simulink model "empirical_cell_twaice_balancing"  (R2024b)
settings: Solver=FixedStepAuto  StartTime=0.0  StopTime=inf  FixedStep=1  RelTol=1e-3
values from neighbouring files (symbols this model uses):
  act = 1    [RunMe_TWAICE_Cell_Model_Farasis_P75_75Ah_v8_1_3.m]
  lic_no = fin_convert(Prod_lic)    [RunMe_TWAICE_Cell_Model_Farasis_P75_75Ah_v8_1_3.m]
  Ts = 1    [RunMe_TWAICE_Cell_Model_Farasis_P75_75Ah_v8_1_3.m]
undefined symbols (not defined in the file or in its folder): DWORK0, DWORK1, DWORK10, DWORK11, DWORK12, DWORK13, DWORK14, DWORK15, DWORK16, DWORK17, DWORK18, DWORK19, DWORK2, DWORK20, DWORK22, DWORK23, DWORK24, DWORK25, DWORK26, DWORK27, DWORK28, DWORK29, DWORK3, DWORK30, DWORK31, DWORK32, DWORK33, DWORK34, DWORK35, DWORK36, DWORK4, DWORK5, DWORK6, DWORK7, DWORK8, DWORK9, SOHc_init, SOHr_init
libraries: fl_lib x73, nesl_utility x32, ee_lib x8
(part 3 of 4)

== system empirical_cell_twaice_balancing/Cell 5/ETA Model 1 ==
  "Current " : Inport  OutDataTypeStr=double  PortDimensions=1
  T_ambient / °C : Inport  Port=2  OutDataTypeStr=double  PortDimensions=1
  SOHc_init : Inport  Port=3
  SOHr_init : Inport  Port=4
  SOC_init : Inport  Port=5
  T_init : Inport  Port=6
  SOC_in : Inport  Port=7
  SOH : Inport  Port=8
  ETA Model _sfcn : S-Function  FunctionName=ETA_sf  Parameters=sfcnParam1, sfcnParam2, sfcnParam3  SFunctionModules=""  SFunctionDeploymentMode=off  EnableBusSupport=off  SFcnStateName=DWORK0,DWORK1,DWORK2,DWORK3,DWORK4,DWORK5,DWORK6,DWORK7,DWORK8,DWORK9,DWORK10,DWORK11,DWORK12,DWORK13,DWORK14,DWORK15,DWORK16,DWORK17,DWORK18,DWORK19,DWORK20,DWORK22,DWORK23,DWORK24,DWORK25,DWORK26,DWORK27,DWORK28,DWORK29,DWORK30,DWORK31,DWORK32,DWORK33,DWORK34,DWORK35,DWORK36  mask{rtw_sf_name=ETA_sf, showVar=off, sfcnParam1=sfcnParam1, sfcnParam2=sfcnParam2, sfcnParam3=sfcnParam3}
      mask prompts: rtw_sf_name "Simulink:masks:GenSFuncName_MP"; showVar "Simulink:masks:GenSFuncShowModuleList_MP"; sfcnParam1 "Ts:"; sfcnParam2 "act:"; sfcnParam3 "lic_no:"
      mask help: Simulink:masks:GenSFuncDesc_MD
      mask init: same as empirical_cell_twaice_balancing/Cell 1/ETA Model 1/ETA Model _sfcn
      settings: SFcnIsStateOwnerBlock=on
      settings: CopyFcn=|
      | if ~strcmp(get_param(gcb,'Linkstatus'),'none') && ...
      | ~strcmp(get_param(gcb,'Linkstatus'),'implicit')
      |   set_param(gcb,'LinkStatus','none');
      | end
      mask Help: eval('feval(''rtwprivate'',''rtwhelpview'',''rtw_sfcn_block'')');
      mask Display:
      | port_label('input',1,'Current ');
      | port_label('input',2,'T_ambient / °C');
      | port_label('input',3,'htc_in');
      | port_label('input',4,'Pcool_in');
      | port_label('input',5,'SOHc_init');
      | port_label('input',6,'SOHr_init');
      | port_label('input',7,'SOC_init');
      | port_label('input',8,'T_init');
      | port_label('input',9,'SOC_in');
      | port_label('input',10,'SOHc');
      | port_label('input',11,'SOHr');
      | port_label('output',1,'Current / A');
      | port_label('output',2,'Voltage / V');
      | port_label('output',3,'SOC / 0..1');
      | port_label('output',4,'SOHc / 0..1');
      | port_label('output',5,'T_sim / °C');
      | port_label('output',6,'Generated Heat / W');
      | port_label('output',7,'SOHr / 1');
      | port_label('output',8,'Power_sim / W');
      | port_label('output',9,'total_Ah');
  __InputSSForSFun__ : Subsystem
  __OutputSSForSFun__ : Subsystem
  Current / A : Outport  OutDataTypeStr=double  PortDimensions=1
  Voltage / V : Outport  Port=2  OutDataTypeStr=double  PortDimensions=1
  SOC / 0..1 : Outport  Port=3  OutDataTypeStr=double  PortDimensions=1
  SOHc / 0..1 : Outport  Port=4  OutDataTypeStr=double  PortDimensions=1
  T_sim / °C : Outport  Port=5  OutDataTypeStr=double  PortDimensions=1
  Generated Heat / W : Outport  Port=6  OutDataTypeStr=double  PortDimensions=1
  SOHr / 1 : Outport  Port=7  OutDataTypeStr=double  PortDimensions=1
  Power_sim / W : Outport  Port=8  OutDataTypeStr=double  PortDimensions=1
  total_Ah : Outport  Port=9
  wires:
  "Current "/1 -> __InputSSForSFun__/1("Current ")
  T_ambient / °C/1 -> __InputSSForSFun__/2(T_ambient / °C)
  SOHc_init/1 -> __InputSSForSFun__/3(SOHc_init)
  SOHr_init/1 -> __InputSSForSFun__/4(SOHr_init)
  SOC_init/1 -> __InputSSForSFun__/5(SOC_init)
  T_init/1 -> __InputSSForSFun__/6(T_init)
  SOC_in/1 -> __InputSSForSFun__/7(SOC_in)
  SOH/1 -> __InputSSForSFun__/8(SOH)
  __InputSSForSFun__/1(__UniqueOutportName__1__) -> ETA Model _sfcn/1
  __InputSSForSFun__/2(__UniqueOutportName__2__) -> ETA Model _sfcn/2
  __InputSSForSFun__/3(__UniqueOutportName__3__) -> ETA Model _sfcn/3
  __InputSSForSFun__/4(__UniqueOutportName__4__) -> ETA Model _sfcn/4
  __InputSSForSFun__/5(__UniqueOutportName__5__) -> ETA Model _sfcn/5
  __InputSSForSFun__/6(__UniqueOutportName__6__) -> ETA Model _sfcn/6
  __InputSSForSFun__/7(__UniqueOutportName__7__) -> ETA Model _sfcn/7
  __InputSSForSFun__/8(__UniqueOutportName__8__) -> ETA Model _sfcn/8
  __InputSSForSFun__/9(__UniqueOutportName__9__) -> ETA Model _sfcn/9
  __InputSSForSFun__/10(__UniqueOutportName__10__) -> ETA Model _sfcn/10
  __InputSSForSFun__/11(__UniqueOutportName__11__) -> ETA Model _sfcn/11
  ETA Model _sfcn/1 -> __OutputSSForSFun__/1(__UniqueInportName__1__)
  ETA Model _sfcn/2 -> __OutputSSForSFun__/2(__UniqueInportName__2__)
  ETA Model _sfcn/3 -> __OutputSSForSFun__/3(__UniqueInportName__3__)
  ETA Model _sfcn/4 -> __OutputSSForSFun__/4(__UniqueInportName__4__)
  ETA Model _sfcn/5 -> __OutputSSForSFun__/5(__UniqueInportName__5__)
  ETA Model _sfcn/6 -> __OutputSSForSFun__/6(__UniqueInportName__6__)
  ETA Model _sfcn/7 -> __OutputSSForSFun__/7(__UniqueInportName__7__)
  ETA Model _sfcn/8 -> __OutputSSForSFun__/8(__UniqueInportName__8__)
  ETA Model _sfcn/9 -> __OutputSSForSFun__/9(__UniqueInportName__9__)
  __OutputSSForSFun__/1(Current / A) -> Current / A/1
  __OutputSSForSFun__/2(Voltage / V) -> Voltage / V/1
  __OutputSSForSFun__/3(SOC / 0..1) -> SOC / 0..1/1
  __OutputSSForSFun__/4(SOHc / 0..1) -> SOHc / 0..1/1
  __OutputSSForSFun__/5(T_sim / °C) -> T_sim / °C/1
  __OutputSSForSFun__/6(Generated Heat / W) -> Generated Heat / W/1
  __OutputSSForSFun__/7(SOHr / 1) -> SOHr / 1/1
  __OutputSSForSFun__/8(Power_sim / W) -> Power_sim / W/1
  __OutputSSForSFun__/9(total_Ah) -> total_Ah/1

== system empirical_cell_twaice_balancing/Cell 5/SOC coloumb counting1 ==
  SOC_init : Inport
  T_init : Inport  Port=2
  I [A] : Inport  Port=3
  SOHc : Inport  Port=4
  Tcell : Inport  Port=5
  SOC coloumb counting_sfcn : S-Function  FunctionName=SOC_sf  Parameters=sfcnParam1  SFunctionModules=""  SFunctionDeploymentMode=off  EnableBusSupport=off  SFcnStateName=DWORK0,DWORK1  mask{rtw_sf_name=SOC_sf, showVar=off, sfcnParam1=sfcnParam1}
      mask prompts: rtw_sf_name "Simulink:masks:GenSFuncName_MP"; showVar "Simulink:masks:GenSFuncShowModuleList_MP"; sfcnParam1 "Ts:"
      mask help: Simulink:masks:GenSFuncDesc_MD
      mask init: same as empirical_cell_twaice_balancing/Cell 1/ETA Model 1/ETA Model _sfcn
      settings: SFcnIsStateOwnerBlock=on
      settings: CopyFcn=|
      | if ~strcmp(get_param(gcb,'Linkstatus'),'none') && ...
      | ~strcmp(get_param(gcb,'Linkstatus'),'implicit')
      |   set_param(gcb,'LinkStatus','none');
      | end
      mask Help: eval('feval(''rtwprivate'',''rtwhelpview'',''rtw_sfcn_block'')');
      mask Display:
      | port_label('input',1,'SOC_init');
      | port_label('input',2,'T_init');
      | port_label('input',3,'I [A]');
      | port_label('input',4,'SOHc');
      | port_label('input',5,'Tcell');
      | port_label('output',1,'SOC');
  __InputSSForSFun__ : Subsystem
  __OutputSSForSFun__ : Subsystem
  SOC : Outport  VectorParamsAs1DForOutWhenUnconnected=off
  wires:
  SOC_init/1 -> __InputSSForSFun__/1(SOC_init)
  T_init/1 -> __InputSSForSFun__/2(T_init)
  I [A]/1 -> __InputSSForSFun__/3(I [A])
  SOHc/1 -> __InputSSForSFun__/4(SOHc)
  Tcell/1 -> __InputSSForSFun__/5(Tcell)
  __InputSSForSFun__/1(__UniqueOutportName__1__) -> SOC coloumb counting_sfcn/1
  __InputSSForSFun__/2(__UniqueOutportName__2__) -> SOC coloumb counting_sfcn/2
  __InputSSForSFun__/3(__UniqueOutportName__3__) -> SOC coloumb counting_sfcn/3
  __InputSSForSFun__/4(__UniqueOutportName__4__) -> SOC coloumb counting_sfcn/4
  __InputSSForSFun__/5(__UniqueOutportName__5__) -> SOC coloumb counting_sfcn/5
  SOC coloumb counting_sfcn/1 -> __OutputSSForSFun__/1(__UniqueInportName__1__)
  __OutputSSForSFun__/1(SOC) -> SOC/1

== system empirical_cell_twaice_balancing/Cell 6/ETA Model 1 ==
  "Current " : Inport  OutDataTypeStr=double  PortDimensions=1
  T_ambient / °C : Inport  Port=2  OutDataTypeStr=double  PortDimensions=1
  SOHc_init : Inport  Port=3
  SOHr_init : Inport  Port=4
  SOC_init : Inport  Port=5
  T_init : Inport  Port=6
  SOC_in : Inport  Port=7
  SOH : Inport  Port=8
  ETA Model _sfcn : S-Function  FunctionName=ETA_sf  Parameters=sfcnParam1, sfcnParam2, sfcnParam3  SFunctionModules=""  SFunctionDeploymentMode=off  EnableBusSupport=off  SFcnStateName=DWORK0,DWORK1,DWORK2,DWORK3,DWORK4,DWORK5,DWORK6,DWORK7,DWORK8,DWORK9,DWORK10,DWORK11,DWORK12,DWORK13,DWORK14,DWORK15,DWORK16,DWORK17,DWORK18,DWORK19,DWORK20,DWORK22,DWORK23,DWORK24,DWORK25,DWORK26,DWORK27,DWORK28,DWORK29,DWORK30,DWORK31,DWORK32,DWORK33,DWORK34,DWORK35,DWORK36  mask{rtw_sf_name=ETA_sf, showVar=off, sfcnParam1=sfcnParam1, sfcnParam2=sfcnParam2, sfcnParam3=sfcnParam3}
      mask prompts: rtw_sf_name "Simulink:masks:GenSFuncName_MP"; showVar "Simulink:masks:GenSFuncShowModuleList_MP"; sfcnParam1 "Ts:"; sfcnParam2 "act:"; sfcnParam3 "lic_no:"
      mask help: Simulink:masks:GenSFuncDesc_MD
      mask init: same as empirical_cell_twaice_balancing/Cell 1/ETA Model 1/ETA Model _sfcn
      settings: SFcnIsStateOwnerBlock=on
      settings: CopyFcn=|
      | if ~strcmp(get_param(gcb,'Linkstatus'),'none') && ...
      | ~strcmp(get_param(gcb,'Linkstatus'),'implicit')
      |   set_param(gcb,'LinkStatus','none');
      | end
      mask Help: eval('feval(''rtwprivate'',''rtwhelpview'',''rtw_sfcn_block'')');
      mask Display:
      | port_label('input',1,'Current ');
      | port_label('input',2,'T_ambient / °C');
      | port_label('input',3,'htc_in');
      | port_label('input',4,'Pcool_in');
      | port_label('input',5,'SOHc_init');
      | port_label('input',6,'SOHr_init');
      | port_label('input',7,'SOC_init');
      | port_label('input',8,'T_init');
      | port_label('input',9,'SOC_in');
      | port_label('input',10,'SOHc');
      | port_label('input',11,'SOHr');
      | port_label('output',1,'Current / A');
      | port_label('output',2,'Voltage / V');
      | port_label('output',3,'SOC / 0..1');
      | port_label('output',4,'SOHc / 0..1');
      | port_label('output',5,'T_sim / °C');
      | port_label('output',6,'Generated Heat / W');
      | port_label('output',7,'SOHr / 1');
      | port_label('output',8,'Power_sim / W');
      | port_label('output',9,'total_Ah');
  __InputSSForSFun__ : Subsystem
  __OutputSSForSFun__ : Subsystem
  Current / A : Outport  OutDataTypeStr=double  PortDimensions=1
  Voltage / V : Outport  Port=2  OutDataTypeStr=double  PortDimensions=1
  SOC / 0..1 : Outport  Port=3  OutDataTypeStr=double  PortDimensions=1
  SOHc / 0..1 : Outport  Port=4  OutDataTypeStr=double  PortDimensions=1
  T_sim / °C : Outport  Port=5  OutDataTypeStr=double  PortDimensions=1
  Generated Heat / W : Outport  Port=6  OutDataTypeStr=double  PortDimensions=1
  SOHr / 1 : Outport  Port=7  OutDataTypeStr=double  PortDimensions=1
  Power_sim / W : Outport  Port=8  OutDataTypeStr=double  PortDimensions=1
  total_Ah : Outport  Port=9
  wires:
  "Current "/1 -> __InputSSForSFun__/1("Current ")
  T_ambient / °C/1 -> __InputSSForSFun__/2(T_ambient / °C)
  SOHc_init/1 -> __InputSSForSFun__/3(SOHc_init)
  SOHr_init/1 -> __InputSSForSFun__/4(SOHr_init)
  SOC_init/1 -> __InputSSForSFun__/5(SOC_init)
  T_init/1 -> __InputSSForSFun__/6(T_init)
  SOC_in/1 -> __InputSSForSFun__/7(SOC_in)
  SOH/1 -> __InputSSForSFun__/8(SOH)
  __InputSSForSFun__/1(__UniqueOutportName__1__) -> ETA Model _sfcn/1
  __InputSSForSFun__/2(__UniqueOutportName__2__) -> ETA Model _sfcn/2
  __InputSSForSFun__/3(__UniqueOutportName__3__) -> ETA Model _sfcn/3
  __InputSSForSFun__/4(__UniqueOutportName__4__) -> ETA Model _sfcn/4
  __InputSSForSFun__/5(__UniqueOutportName__5__) -> ETA Model _sfcn/5
  __InputSSForSFun__/6(__UniqueOutportName__6__) -> ETA Model _sfcn/6
  __InputSSForSFun__/7(__UniqueOutportName__7__) -> ETA Model _sfcn/7
  __InputSSForSFun__/8(__UniqueOutportName__8__) -> ETA Model _sfcn/8
  __InputSSForSFun__/9(__UniqueOutportName__9__) -> ETA Model _sfcn/9
  __InputSSForSFun__/10(__UniqueOutportName__10__) -> ETA Model _sfcn/10
  __InputSSForSFun__/11(__UniqueOutportName__11__) -> ETA Model _sfcn/11
  ETA Model _sfcn/1 -> __OutputSSForSFun__/1(__UniqueInportName__1__)
  ETA Model _sfcn/2 -> __OutputSSForSFun__/2(__UniqueInportName__2__)
  ETA Model _sfcn/3 -> __OutputSSForSFun__/3(__UniqueInportName__3__)
  ETA Model _sfcn/4 -> __OutputSSForSFun__/4(__UniqueInportName__4__)
  ETA Model _sfcn/5 -> __OutputSSForSFun__/5(__UniqueInportName__5__)
  ETA Model _sfcn/6 -> __OutputSSForSFun__/6(__UniqueInportName__6__)
  ETA Model _sfcn/7 -> __OutputSSForSFun__/7(__UniqueInportName__7__)
  ETA Model _sfcn/8 -> __OutputSSForSFun__/8(__UniqueInportName__8__)
  ETA Model _sfcn/9 -> __OutputSSForSFun__/9(__UniqueInportName__9__)
  __OutputSSForSFun__/1(Current / A) -> Current / A/1
  __OutputSSForSFun__/2(Voltage / V) -> Voltage / V/1
  __OutputSSForSFun__/3(SOC / 0..1) -> SOC / 0..1/1
  __OutputSSForSFun__/4(SOHc / 0..1) -> SOHc / 0..1/1
  __OutputSSForSFun__/5(T_sim / °C) -> T_sim / °C/1
  __OutputSSForSFun__/6(Generated Heat / W) -> Generated Heat / W/1
  __OutputSSForSFun__/7(SOHr / 1) -> SOHr / 1/1
  __OutputSSForSFun__/8(Power_sim / W) -> Power_sim / W/1
  __OutputSSForSFun__/9(total_Ah) -> total_Ah/1

== system empirical_cell_twaice_balancing/Cell 6/SOC coloumb counting1 ==
  SOC_init : Inport
  T_init : Inport  Port=2
  I [A] : Inport  Port=3
  SOHc : Inport  Port=4
  Tcell : Inport  Port=5
  SOC coloumb counting_sfcn : S-Function  FunctionName=SOC_sf  Parameters=sfcnParam1  SFunctionModules=""  SFunctionDeploymentMode=off  EnableBusSupport=off  SFcnStateName=DWORK0,DWORK1  mask{rtw_sf_name=SOC_sf, showVar=off, sfcnParam1=sfcnParam1}
      mask prompts: rtw_sf_name "Simulink:masks:GenSFuncName_MP"; showVar "Simulink:masks:GenSFuncShowModuleList_MP"; sfcnParam1 "Ts:"
      mask help: Simulink:masks:GenSFuncDesc_MD
      mask init: same as empirical_cell_twaice_balancing/Cell 1/ETA Model 1/ETA Model _sfcn
      settings: SFcnIsStateOwnerBlock=on
      settings: CopyFcn=|
      | if ~strcmp(get_param(gcb,'Linkstatus'),'none') && ...
      | ~strcmp(get_param(gcb,'Linkstatus'),'implicit')
      |   set_param(gcb,'LinkStatus','none');
      | end
      mask Help: eval('feval(''rtwprivate'',''rtwhelpview'',''rtw_sfcn_block'')');
      mask Display:
      | port_label('input',1,'SOC_init');
      | port_label('input',2,'T_init');
      | port_label('input',3,'I [A]');
      | port_label('input',4,'SOHc');
      | port_label('input',5,'Tcell');
      | port_label('output',1,'SOC');
  __InputSSForSFun__ : Subsystem
  __OutputSSForSFun__ : Subsystem
  SOC : Outport  VectorParamsAs1DForOutWhenUnconnected=off
  wires:
  SOC_init/1 -> __InputSSForSFun__/1(SOC_init)
  T_init/1 -> __InputSSForSFun__/2(T_init)
  I [A]/1 -> __InputSSForSFun__/3(I [A])
  SOHc/1 -> __InputSSForSFun__/4(SOHc)
  Tcell/1 -> __InputSSForSFun__/5(Tcell)
  __InputSSForSFun__/1(__UniqueOutportName__1__) -> SOC coloumb counting_sfcn/1
  __InputSSForSFun__/2(__UniqueOutportName__2__) -> SOC coloumb counting_sfcn/2
  __InputSSForSFun__/3(__UniqueOutportName__3__) -> SOC coloumb counting_sfcn/3
  __InputSSForSFun__/4(__UniqueOutportName__4__) -> SOC coloumb counting_sfcn/4
  __InputSSForSFun__/5(__UniqueOutportName__5__) -> SOC coloumb counting_sfcn/5
  SOC coloumb counting_sfcn/1 -> __OutputSSForSFun__/1(__UniqueInportName__1__)
  __OutputSSForSFun__/1(SOC) -> SOC/1

== system empirical_cell_twaice_balancing/Cell 7/ETA Model 1 ==
  "Current " : Inport  OutDataTypeStr=double  PortDimensions=1
  T_ambient / °C : Inport  Port=2  OutDataTypeStr=double  PortDimensions=1
  SOHc_init : Inport  Port=3
  SOHr_init : Inport  Port=4
  SOC_init : Inport  Port=5
  T_init : Inport  Port=6
  SOC_in : Inport  Port=7
  SOH : Inport  Port=8
  ETA Model _sfcn : S-Function  FunctionName=ETA_sf  Parameters=sfcnParam1, sfcnParam2, sfcnParam3  SFunctionModules=""  SFunctionDeploymentMode=off  EnableBusSupport=off  SFcnStateName=DWORK0,DWORK1,DWORK2,DWORK3,DWORK4,DWORK5,DWORK6,DWORK7,DWORK8,DWORK9,DWORK10,DWORK11,DWORK12,DWORK13,DWORK14,DWORK15,DWORK16,DWORK17,DWORK18,DWORK19,DWORK20,DWORK22,DWORK23,DWORK24,DWORK25,DWORK26,DWORK27,DWORK28,DWORK29,DWORK30,DWORK31,DWORK32,DWORK33,DWORK34,DWORK35,DWORK36  mask{rtw_sf_name=ETA_sf, showVar=off, sfcnParam1=sfcnParam1, sfcnParam2=sfcnParam2, sfcnParam3=sfcnParam3}
      mask prompts: rtw_sf_name "Simulink:masks:GenSFuncName_MP"; showVar "Simulink:masks:GenSFuncShowModuleList_MP"; sfcnParam1 "Ts:"; sfcnParam2 "act:"; sfcnParam3 "lic_no:"
      mask help: Simulink:masks:GenSFuncDesc_MD
      mask init: same as empirical_cell_twaice_balancing/Cell 1/ETA Model 1/ETA Model _sfcn
      settings: SFcnIsStateOwnerBlock=on
      settings: CopyFcn=|
      | if ~strcmp(get_param(gcb,'Linkstatus'),'none') && ...
      | ~strcmp(get_param(gcb,'Linkstatus'),'implicit')
      |   set_param(gcb,'LinkStatus','none');
      | end
      mask Help: eval('feval(''rtwprivate'',''rtwhelpview'',''rtw_sfcn_block'')');
      mask Display:
      | port_label('input',1,'Current ');
      | port_label('input',2,'T_ambient / °C');
      | port_label('input',3,'htc_in');
      | port_label('input',4,'Pcool_in');
      | port_label('input',5,'SOHc_init');
      | port_label('input',6,'SOHr_init');
      | port_label('input',7,'SOC_init');
      | port_label('input',8,'T_init');
      | port_label('input',9,'SOC_in');
      | port_label('input',10,'SOHc');
      | port_label('input',11,'SOHr');
      | port_label('output',1,'Current / A');
      | port_label('output',2,'Voltage / V');
      | port_label('output',3,'SOC / 0..1');
      | port_label('output',4,'SOHc / 0..1');
      | port_label('output',5,'T_sim / °C');
      | port_label('output',6,'Generated Heat / W');
      | port_label('output',7,'SOHr / 1');
      | port_label('output',8,'Power_sim / W');
      | port_label('output',9,'total_Ah');
  __InputSSForSFun__ : Subsystem
  __OutputSSForSFun__ : Subsystem
  Current / A : Outport  OutDataTypeStr=double  PortDimensions=1
  Voltage / V : Outport  Port=2  OutDataTypeStr=double  PortDimensions=1
  SOC / 0..1 : Outport  Port=3  OutDataTypeStr=double  PortDimensions=1
  SOHc / 0..1 : Outport  Port=4  OutDataTypeStr=double  PortDimensions=1
  T_sim / °C : Outport  Port=5  OutDataTypeStr=double  PortDimensions=1
  Generated Heat / W : Outport  Port=6  OutDataTypeStr=double  PortDimensions=1
  SOHr / 1 : Outport  Port=7  OutDataTypeStr=double  PortDimensions=1
  Power_sim / W : Outport  Port=8  OutDataTypeStr=double  PortDimensions=1
  total_Ah : Outport  Port=9
  wires:
  "Current "/1 -> __InputSSForSFun__/1("Current ")
  T_ambient / °C/1 -> __InputSSForSFun__/2(T_ambient / °C)
  SOHc_init/1 -> __InputSSForSFun__/3(SOHc_init)
  SOHr_init/1 -> __InputSSForSFun__/4(SOHr_init)
  SOC_init/1 -> __InputSSForSFun__/5(SOC_init)
  T_init/1 -> __InputSSForSFun__/6(T_init)
  SOC_in/1 -> __InputSSForSFun__/7(SOC_in)
  SOH/1 -> __InputSSForSFun__/8(SOH)
  __InputSSForSFun__/1(__UniqueOutportName__1__) -> ETA Model _sfcn/1
  __InputSSForSFun__/2(__UniqueOutportName__2__) -> ETA Model _sfcn/2
  __InputSSForSFun__/3(__UniqueOutportName__3__) -> ETA Model _sfcn/3
  __InputSSForSFun__/4(__UniqueOutportName__4__) -> ETA Model _sfcn/4
  __InputSSForSFun__/5(__UniqueOutportName__5__) -> ETA Model _sfcn/5
  __InputSSForSFun__/6(__UniqueOutportName__6__) -> ETA Model _sfcn/6
  __InputSSForSFun__/7(__UniqueOutportName__7__) -> ETA Model _sfcn/7
  __InputSSForSFun__/8(__UniqueOutportName__8__) -> ETA Model _sfcn/8
  __InputSSForSFun__/9(__UniqueOutportName__9__) -> ETA Model _sfcn/9
  __InputSSForSFun__/10(__UniqueOutportName__10__) -> ETA Model _sfcn/10
  __InputSSForSFun__/11(__UniqueOutportName__11__) -> ETA Model _sfcn/11
  ETA Model _sfcn/1 -> __OutputSSForSFun__/1(__UniqueInportName__1__)
  ETA Model _sfcn/2 -> __OutputSSForSFun__/2(__UniqueInportName__2__)
  ETA Model _sfcn/3 -> __OutputSSForSFun__/3(__UniqueInportName__3__)
  ETA Model _sfcn/4 -> __OutputSSForSFun__/4(__UniqueInportName__4__)
  ETA Model _sfcn/5 -> __OutputSSForSFun__/5(__UniqueInportName__5__)
  ETA Model _sfcn/6 -> __OutputSSForSFun__/6(__UniqueInportName__6__)
  ETA Model _sfcn/7 -> __OutputSSForSFun__/7(__UniqueInportName__7__)
  ETA Model _sfcn/8 -> __OutputSSForSFun__/8(__UniqueInportName__8__)
  ETA Model _sfcn/9 -> __OutputSSForSFun__/9(__UniqueInportName__9__)
  __OutputSSForSFun__/1(Current / A) -> Current / A/1
  __OutputSSForSFun__/2(Voltage / V) -> Voltage / V/1
  __OutputSSForSFun__/3(SOC / 0..1) -> SOC / 0..1/1
  __OutputSSForSFun__/4(SOHc / 0..1) -> SOHc / 0..1/1
  __OutputSSForSFun__/5(T_sim / °C) -> T_sim / °C/1
  __OutputSSForSFun__/6(Generated Heat / W) -> Generated Heat / W/1
  __OutputSSForSFun__/7(SOHr / 1) -> SOHr / 1/1
  __OutputSSForSFun__/8(Power_sim / W) -> Power_sim / W/1
  __OutputSSForSFun__/9(total_Ah) -> total_Ah/1

== system empirical_cell_twaice_balancing/Cell 7/SOC coloumb counting1 ==
  SOC_init : Inport
  T_init : Inport  Port=2
  I [A] : Inport  Port=3
  SOHc : Inport  Port=4
  Tcell : Inport  Port=5
  SOC coloumb counting_sfcn : S-Function  FunctionName=SOC_sf  Parameters=sfcnParam1  SFunctionModules=""  SFunctionDeploymentMode=off  EnableBusSupport=off  SFcnStateName=DWORK0,DWORK1  mask{rtw_sf_name=SOC_sf, showVar=off, sfcnParam1=sfcnParam1}
      mask prompts: rtw_sf_name "Simulink:masks:GenSFuncName_MP"; showVar "Simulink:masks:GenSFuncShowModuleList_MP"; sfcnParam1 "Ts:"
      mask help: Simulink:masks:GenSFuncDesc_MD
      mask init: same as empirical_cell_twaice_balancing/Cell 1/ETA Model 1/ETA Model _sfcn
      settings: SFcnIsStateOwnerBlock=on
      settings: CopyFcn=|
      | if ~strcmp(get_param(gcb,'Linkstatus'),'none') && ...
      | ~strcmp(get_param(gcb,'Linkstatus'),'implicit')
      |   set_param(gcb,'LinkStatus','none');
      | end
      mask Help: eval('feval(''rtwprivate'',''rtwhelpview'',''rtw_sfcn_block'')');
      mask Display:
      | port_label('input',1,'SOC_init');
      | port_label('input',2,'T_init');
      | port_label('input',3,'I [A]');
      | port_label('input',4,'SOHc');
      | port_label('input',5,'Tcell');
      | port_label('output',1,'SOC');
  __InputSSForSFun__ : Subsystem
  __OutputSSForSFun__ : Subsystem
  SOC : Outport  VectorParamsAs1DForOutWhenUnconnected=off
  wires:
  SOC_init/1 -> __InputSSForSFun__/1(SOC_init)
  T_init/1 -> __InputSSForSFun__/2(T_init)
  I [A]/1 -> __InputSSForSFun__/3(I [A])
  SOHc/1 -> __InputSSForSFun__/4(SOHc)
  Tcell/1 -> __InputSSForSFun__/5(Tcell)
  __InputSSForSFun__/1(__UniqueOutportName__1__) -> SOC coloumb counting_sfcn/1
  __InputSSForSFun__/2(__UniqueOutportName__2__) -> SOC coloumb counting_sfcn/2
  __InputSSForSFun__/3(__UniqueOutportName__3__) -> SOC coloumb counting_sfcn/3
  __InputSSForSFun__/4(__UniqueOutportName__4__) -> SOC coloumb counting_sfcn/4
  __InputSSForSFun__/5(__UniqueOutportName__5__) -> SOC coloumb counting_sfcn/5
  SOC coloumb counting_sfcn/1 -> __OutputSSForSFun__/1(__UniqueInportName__1__)
  __OutputSSForSFun__/1(SOC) -> SOC/1

== system empirical_cell_twaice_balancing/Cell 8/ETA Model 1 ==
  "Current " : Inport  OutDataTypeStr=double  PortDimensions=1
  T_ambient / °C : Inport  Port=2  OutDataTypeStr=double  PortDimensions=1
  SOHc_init : Inport  Port=3
  SOHr_init : Inport  Port=4
  SOC_init : Inport  Port=5
  T_init : Inport  Port=6
  SOC_in : Inport  Port=7
  SOH : Inport  Port=8
  ETA Model _sfcn : S-Function  FunctionName=ETA_sf  Parameters=sfcnParam1, sfcnParam2, sfcnParam3  SFunctionModules=""  SFunctionDeploymentMode=off  EnableBusSupport=off  SFcnStateName=DWORK0,DWORK1,DWORK2,DWORK3,DWORK4,DWORK5,DWORK6,DWORK7,DWORK8,DWORK9,DWORK10,DWORK11,DWORK12,DWORK13,DWORK14,DWORK15,DWORK16,DWORK17,DWORK18,DWORK19,DWORK20,DWORK22,DWORK23,DWORK24,DWORK25,DWORK26,DWORK27,DWORK28,DWORK29,DWORK30,DWORK31,DWORK32,DWORK33,DWORK34,DWORK35,DWORK36  mask{rtw_sf_name=ETA_sf, showVar=off, sfcnParam1=sfcnParam1, sfcnParam2=sfcnParam2, sfcnParam3=sfcnParam3}
      mask prompts: rtw_sf_name "Simulink:masks:GenSFuncName_MP"; showVar "Simulink:masks:GenSFuncShowModuleList_MP"; sfcnParam1 "Ts:"; sfcnParam2 "act:"; sfcnParam3 "lic_no:"
      mask help: Simulink:masks:GenSFuncDesc_MD
      mask init: same as empirical_cell_twaice_balancing/Cell 1/ETA Model 1/ETA Model _sfcn
      settings: SFcnIsStateOwnerBlock=on
      settings: CopyFcn=|
      | if ~strcmp(get_param(gcb,'Linkstatus'),'none') && ...
      | ~strcmp(get_param(gcb,'Linkstatus'),'implicit')
      |   set_param(gcb,'LinkStatus','none');
      | end
      mask Help: eval('feval(''rtwprivate'',''rtwhelpview'',''rtw_sfcn_block'')');
      mask Display:
      | port_label('input',1,'Current ');
      | port_label('input',2,'T_ambient / °C');
      | port_label('input',3,'htc_in');
      | port_label('input',4,'Pcool_in');
      | port_label('input',5,'SOHc_init');
      | port_label('input',6,'SOHr_init');
      | port_label('input',7,'SOC_init');
      | port_label('input',8,'T_init');
      | port_label('input',9,'SOC_in');
      | port_label('input',10,'SOHc');
      | port_label('input',11,'SOHr');
      | port_label('output',1,'Current / A');
      | port_label('output',2,'Voltage / V');
      | port_label('output',3,'SOC / 0..1');
      | port_label('output',4,'SOHc / 0..1');
      | port_label('output',5,'T_sim / °C');
      | port_label('output',6,'Generated Heat / W');
      | port_label('output',7,'SOHr / 1');
      | port_label('output',8,'Power_sim / W');
      | port_label('output',9,'total_Ah');
  __InputSSForSFun__ : Subsystem
  __OutputSSForSFun__ : Subsystem
  Current / A : Outport  OutDataTypeStr=double  PortDimensions=1
  Voltage / V : Outport  Port=2  OutDataTypeStr=double  PortDimensions=1
  SOC / 0..1 : Outport  Port=3  OutDataTypeStr=double  PortDimensions=1
  SOHc / 0..1 : Outport  Port=4  OutDataTypeStr=double  PortDimensions=1
  T_sim / °C : Outport  Port=5  OutDataTypeStr=double  PortDimensions=1
  Generated Heat / W : Outport  Port=6  OutDataTypeStr=double  PortDimensions=1
  SOHr / 1 : Outport  Port=7  OutDataTypeStr=double  PortDimensions=1
  Power_sim / W : Outport  Port=8  OutDataTypeStr=double  PortDimensions=1
  total_Ah : Outport  Port=9
  wires:
  "Current "/1 -> __InputSSForSFun__/1("Current ")
  T_ambient / °C/1 -> __InputSSForSFun__/2(T_ambient / °C)
  SOHc_init/1 -> __InputSSForSFun__/3(SOHc_init)
  SOHr_init/1 -> __InputSSForSFun__/4(SOHr_init)
  SOC_init/1 -> __InputSSForSFun__/5(SOC_init)
  T_init/1 -> __InputSSForSFun__/6(T_init)
  SOC_in/1 -> __InputSSForSFun__/7(SOC_in)
  SOH/1 -> __InputSSForSFun__/8(SOH)
  __InputSSForSFun__/1(__UniqueOutportName__1__) -> ETA Model _sfcn/1
  __InputSSForSFun__/2(__UniqueOutportName__2__) -> ETA Model _sfcn/2
  __InputSSForSFun__/3(__UniqueOutportName__3__) -> ETA Model _sfcn/3
  __InputSSForSFun__/4(__UniqueOutportName__4__) -> ETA Model _sfcn/4
  __InputSSForSFun__/5(__UniqueOutportName__5__) -> ETA Model _sfcn/5
  __InputSSForSFun__/6(__UniqueOutportName__6__) -> ETA Model _sfcn/6
  __InputSSForSFun__/7(__UniqueOutportName__7__) -> ETA Model _sfcn/7
  __InputSSForSFun__/8(__UniqueOutportName__8__) -> ETA Model _sfcn/8
  __InputSSForSFun__/9(__UniqueOutportName__9__) -> ETA Model _sfcn/9
  __InputSSForSFun__/10(__UniqueOutportName__10__) -> ETA Model _sfcn/10
  __InputSSForSFun__/11(__UniqueOutportName__11__) -> ETA Model _sfcn/11
  ETA Model _sfcn/1 -> __OutputSSForSFun__/1(__UniqueInportName__1__)
  ETA Model _sfcn/2 -> __OutputSSForSFun__/2(__UniqueInportName__2__)
  ETA Model _sfcn/3 -> __OutputSSForSFun__/3(__UniqueInportName__3__)
  ETA Model _sfcn/4 -> __OutputSSForSFun__/4(__UniqueInportName__4__)
  ETA Model _sfcn/5 -> __OutputSSForSFun__/5(__UniqueInportName__5__)
  ETA Model _sfcn/6 -> __OutputSSForSFun__/6(__UniqueInportName__6__)
  ETA Model _sfcn/7 -> __OutputSSForSFun__/7(__UniqueInportName__7__)
  ETA Model _sfcn/8 -> __OutputSSForSFun__/8(__UniqueInportName__8__)
  ETA Model _sfcn/9 -> __OutputSSForSFun__/9(__UniqueInportName__9__)
  __OutputSSForSFun__/1(Current / A) -> Current / A/1
  __OutputSSForSFun__/2(Voltage / V) -> Voltage / V/1
  __OutputSSForSFun__/3(SOC / 0..1) -> SOC / 0..1/1
  __OutputSSForSFun__/4(SOHc / 0..1) -> SOHc / 0..1/1
  __OutputSSForSFun__/5(T_sim / °C) -> T_sim / °C/1
  __OutputSSForSFun__/6(Generated Heat / W) -> Generated Heat / W/1
  __OutputSSForSFun__/7(SOHr / 1) -> SOHr / 1/1
  __OutputSSForSFun__/8(Power_sim / W) -> Power_sim / W/1
  __OutputSSForSFun__/9(total_Ah) -> total_Ah/1

== system empirical_cell_twaice_balancing/Cell 8/SOC coloumb counting1 ==
  SOC_init : Inport
  T_init : Inport  Port=2
  I [A] : Inport  Port=3
  SOHc : Inport  Port=4
  Tcell : Inport  Port=5
  SOC coloumb counting_sfcn : S-Function  FunctionName=SOC_sf  Parameters=sfcnParam1  SFunctionModules=""  SFunctionDeploymentMode=off  EnableBusSupport=off  SFcnStateName=DWORK0,DWORK1  mask{rtw_sf_name=SOC_sf, showVar=off, sfcnParam1=sfcnParam1}
      mask prompts: rtw_sf_name "Simulink:masks:GenSFuncName_MP"; showVar "Simulink:masks:GenSFuncShowModuleList_MP"; sfcnParam1 "Ts:"
      mask help: Simulink:masks:GenSFuncDesc_MD
      mask init: same as empirical_cell_twaice_balancing/Cell 1/ETA Model 1/ETA Model _sfcn
      settings: SFcnIsStateOwnerBlock=on
      settings: CopyFcn=|
      | if ~strcmp(get_param(gcb,'Linkstatus'),'none') && ...
      | ~strcmp(get_param(gcb,'Linkstatus'),'implicit')
      |   set_param(gcb,'LinkStatus','none');
      | end
      mask Help: eval('feval(''rtwprivate'',''rtwhelpview'',''rtw_sfcn_block'')');
      mask Display:
      | port_label('input',1,'SOC_init');
      | port_label('input',2,'T_init');
      | port_label('input',3,'I [A]');
      | port_label('input',4,'SOHc');
      | port_label('input',5,'Tcell');
      | port_label('output',1,'SOC');
  __InputSSForSFun__ : Subsystem
  __OutputSSForSFun__ : Subsystem
  SOC : Outport  VectorParamsAs1DForOutWhenUnconnected=off
  wires:
  SOC_init/1 -> __InputSSForSFun__/1(SOC_init)
  T_init/1 -> __InputSSForSFun__/2(T_init)
  I [A]/1 -> __InputSSForSFun__/3(I [A])
  SOHc/1 -> __InputSSForSFun__/4(SOHc)
  Tcell/1 -> __InputSSForSFun__/5(Tcell)
  __InputSSForSFun__/1(__UniqueOutportName__1__) -> SOC coloumb counting_sfcn/1
  __InputSSForSFun__/2(__UniqueOutportName__2__) -> SOC coloumb counting_sfcn/2
  __InputSSForSFun__/3(__UniqueOutportName__3__) -> SOC coloumb counting_sfcn/3
  __InputSSForSFun__/4(__UniqueOutportName__4__) -> SOC coloumb counting_sfcn/4
  __InputSSForSFun__/5(__UniqueOutportName__5__) -> SOC coloumb counting_sfcn/5
  SOC coloumb counting_sfcn/1 -> __OutputSSForSFun__/1(__UniqueInportName__1__)
  __OutputSSForSFun__/1(SOC) -> SOC/1

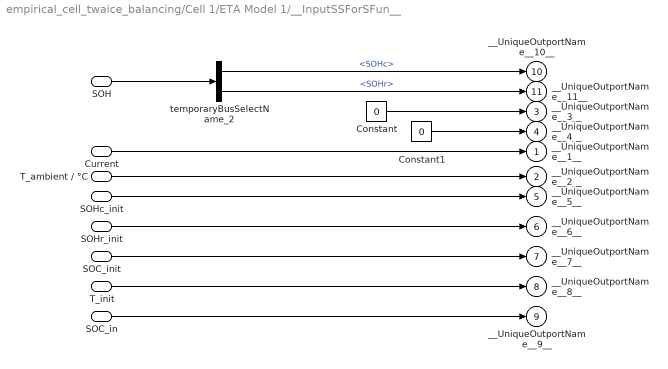
== system empirical_cell_twaice_balancing/Cell 1/ETA Model 1/__InputSSForSFun__ ==
  "Current " : Inport  OutDataTypeStr=double  PortDimensions=1
  T_ambient / °C : Inport  Port=2  OutDataTypeStr=double  PortDimensions=1
  SOHc_init : Inport  Port=3
  SOHr_init : Inport  Port=4
  SOC_init : Inport  Port=5
  T_init : Inport  Port=6
  SOC_in : Inport  Port=7
  SOH : Inport  Port=8
  Constant : Constant  Value=0
  Constant1 : Constant  Value=0
  temporaryBusSelectName_2 : BusSelector  OutputSignals=SOHc,SOHr
  __UniqueOutportName__1__ : Outport  VectorParamsAs1DForOutWhenUnconnected=off
  __UniqueOutportName__2__ : Outport  Port=2  VectorParamsAs1DForOutWhenUnconnected=off
  __UniqueOutportName__3__ : Outport  Port=3  VectorParamsAs1DForOutWhenUnconnected=off
  __UniqueOutportName__4__ : Outport  Port=4  VectorParamsAs1DForOutWhenUnconnected=off
  __UniqueOutportName__5__ : Outport  Port=5  VectorParamsAs1DForOutWhenUnconnected=off
  __UniqueOutportName__6__ : Outport  Port=6  VectorParamsAs1DForOutWhenUnconnected=off
  __UniqueOutportName__7__ : Outport  Port=7  VectorParamsAs1DForOutWhenUnconnected=off
  __UniqueOutportName__8__ : Outport  Port=8  VectorParamsAs1DForOutWhenUnconnected=off
  __UniqueOutportName__9__ : Outport  Port=9  VectorParamsAs1DForOutWhenUnconnected=off
  __UniqueOutportName__10__ : Outport  Port=10  VectorParamsAs1DForOutWhenUnconnected=off
  __UniqueOutportName__11__ : Outport  Port=11  VectorParamsAs1DForOutWhenUnconnected=off
  wires:
  SOH/1 -> temporaryBusSelectName_2/1
  "Current "/1 -> __UniqueOutportName__1__/1
  T_ambient / °C/1 -> __UniqueOutportName__2__/1
  SOHc_init/1 -> __UniqueOutportName__5__/1
  SOHr_init/1 -> __UniqueOutportName__6__/1
  SOC_init/1 -> __UniqueOutportName__7__/1
  T_init/1 -> __UniqueOutportName__8__/1
  SOC_in/1 -> __UniqueOutportName__9__/1
  temporaryBusSelectName_2/1 -> __UniqueOutportName__10__/1  "<SOHc>"
  temporaryBusSelectName_2/2 -> __UniqueOutportName__11__/1  "<SOHr>"
  Constant/1 -> __UniqueOutportName__3__/1
  Constant1/1 -> __UniqueOutportName__4__/1

== system empirical_cell_twaice_balancing/Cell 1/ETA Model 1/__OutputSSForSFun__ ==
  __UniqueInportName__1__ : Inport
  __UniqueInportName__2__ : Inport  Port=2
  __UniqueInportName__3__ : Inport  Port=3
  __UniqueInportName__4__ : Inport  Port=4
  __UniqueInportName__5__ : Inport  Port=5
  __UniqueInportName__6__ : Inport  Port=6
  __UniqueInportName__7__ : Inport  Port=7
  __UniqueInportName__8__ : Inport  Port=8
  __UniqueInportName__9__ : Inport  Port=9
  Current / A : Outport  OutDataTypeStr=double  PortDimensions=1
  Voltage / V : Outport  Port=2  OutDataTypeStr=double  PortDimensions=1
  SOC / 0..1 : Outport  Port=3  OutDataTypeStr=double  PortDimensions=1
  SOHc / 0..1 : Outport  Port=4  OutDataTypeStr=double  PortDimensions=1
  T_sim / °C : Outport  Port=5  OutDataTypeStr=double  PortDimensions=1
  Generated Heat / W : Outport  Port=6  OutDataTypeStr=double  PortDimensions=1
  SOHr / 1 : Outport  Port=7  OutDataTypeStr=double  PortDimensions=1
  Power_sim / W : Outport  Port=8  OutDataTypeStr=double  PortDimensions=1
  total_Ah : Outport  Port=9
  wires:
  __UniqueInportName__1__/1 -> Current / A/1  "I"
  __UniqueInportName__2__/1 -> Voltage / V/1  "U"
  __UniqueInportName__3__/1 -> SOC / 0..1/1
  __UniqueInportName__4__/1 -> SOHc / 0..1/1  "SOHc"
  __UniqueInportName__5__/1 -> T_sim / °C/1  "simulated Temperature"
  __UniqueInportName__6__/1 -> Generated Heat / W/1
  __UniqueInportName__7__/1 -> SOHr / 1/1  "SOHr"
  __UniqueInportName__8__/1 -> Power_sim / W/1
  __UniqueInportName__9__/1 -> total_Ah/1  "total_Ah"

== system empirical_cell_twaice_balancing/Cell 1/SOC coloumb counting1/__InputSSForSFun__ ==
  SOC_init : Inport
  T_init : Inport  Port=2
  I [A] : Inport  Port=3
  SOHc : Inport  Port=4
  Tcell : Inport  Port=5
  __UniqueOutportName__1__ : Outport  VectorParamsAs1DForOutWhenUnconnected=off
  __UniqueOutportName__2__ : Outport  Port=2  VectorParamsAs1DForOutWhenUnconnected=off
  __UniqueOutportName__3__ : Outport  Port=3  VectorParamsAs1DForOutWhenUnconnected=off
  __UniqueOutportName__4__ : Outport  Port=4  VectorParamsAs1DForOutWhenUnconnected=off
  __UniqueOutportName__5__ : Outport  Port=5  VectorParamsAs1DForOutWhenUnconnected=off
  wires:
  SOC_init/1 -> __UniqueOutportName__1__/1
  T_init/1 -> __UniqueOutportName__2__/1
  I [A]/1 -> __UniqueOutportName__3__/1
  SOHc/1 -> __UniqueOutportName__4__/1
  Tcell/1 -> __UniqueOutportName__5__/1

== system empirical_cell_twaice_balancing/Cell 1/SOC coloumb counting1/__OutputSSForSFun__ ==
  __UniqueInportName__1__ : Inport
  SOC : Outport  VectorParamsAs1DForOutWhenUnconnected=off
  wires:
  __UniqueInportName__1__/1 -> SOC/1

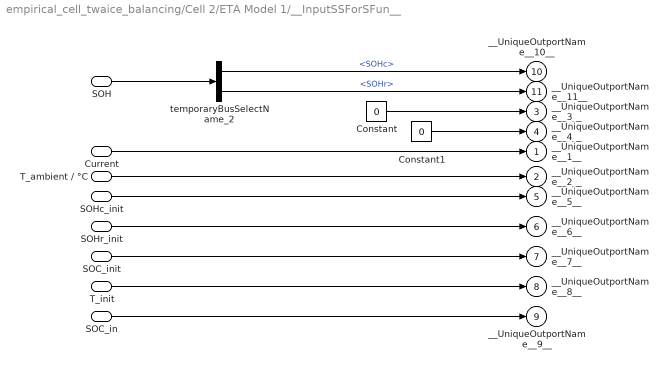
== system empirical_cell_twaice_balancing/Cell 2/ETA Model 1/__InputSSForSFun__ ==
  "Current " : Inport  OutDataTypeStr=double  PortDimensions=1
  T_ambient / °C : Inport  Port=2  OutDataTypeStr=double  PortDimensions=1
  SOHc_init : Inport  Port=3
  SOHr_init : Inport  Port=4
  SOC_init : Inport  Port=5
  T_init : Inport  Port=6
  SOC_in : Inport  Port=7
  SOH : Inport  Port=8
  Constant : Constant  Value=0
  Constant1 : Constant  Value=0
  temporaryBusSelectName_2 : BusSelector  OutputSignals=SOHc,SOHr
  __UniqueOutportName__1__ : Outport  VectorParamsAs1DForOutWhenUnconnected=off
  __UniqueOutportName__2__ : Outport  Port=2  VectorParamsAs1DForOutWhenUnconnected=off
  __UniqueOutportName__3__ : Outport  Port=3  VectorParamsAs1DForOutWhenUnconnected=off
  __UniqueOutportName__4__ : Outport  Port=4  VectorParamsAs1DForOutWhenUnconnected=off
  __UniqueOutportName__5__ : Outport  Port=5  VectorParamsAs1DForOutWhenUnconnected=off
  __UniqueOutportName__6__ : Outport  Port=6  VectorParamsAs1DForOutWhenUnconnected=off
  __UniqueOutportName__7__ : Outport  Port=7  VectorParamsAs1DForOutWhenUnconnected=off
  __UniqueOutportName__8__ : Outport  Port=8  VectorParamsAs1DForOutWhenUnconnected=off
  __UniqueOutportName__9__ : Outport  Port=9  VectorParamsAs1DForOutWhenUnconnected=off
  __UniqueOutportName__10__ : Outport  Port=10  VectorParamsAs1DForOutWhenUnconnected=off
  __UniqueOutportName__11__ : Outport  Port=11  VectorParamsAs1DForOutWhenUnconnected=off
  wires:
  SOH/1 -> temporaryBusSelectName_2/1
  "Current "/1 -> __UniqueOutportName__1__/1
  T_ambient / °C/1 -> __UniqueOutportName__2__/1
  SOHc_init/1 -> __UniqueOutportName__5__/1
  SOHr_init/1 -> __UniqueOutportName__6__/1
  SOC_init/1 -> __UniqueOutportName__7__/1
  T_init/1 -> __UniqueOutportName__8__/1
  SOC_in/1 -> __UniqueOutportName__9__/1
  temporaryBusSelectName_2/1 -> __UniqueOutportName__10__/1  "<SOHc>"
  temporaryBusSelectName_2/2 -> __UniqueOutportName__11__/1  "<SOHr>"
  Constant/1 -> __UniqueOutportName__3__/1
  Constant1/1 -> __UniqueOutportName__4__/1

== system empirical_cell_twaice_balancing/Cell 2/ETA Model 1/__OutputSSForSFun__ ==
  __UniqueInportName__1__ : Inport
  __UniqueInportName__2__ : Inport  Port=2
  __UniqueInportName__3__ : Inport  Port=3
  __UniqueInportName__4__ : Inport  Port=4
  __UniqueInportName__5__ : Inport  Port=5
  __UniqueInportName__6__ : Inport  Port=6
  __UniqueInportName__7__ : Inport  Port=7
  __UniqueInportName__8__ : Inport  Port=8
  __UniqueInportName__9__ : Inport  Port=9
  Current / A : Outport  OutDataTypeStr=double  PortDimensions=1
  Voltage / V : Outport  Port=2  OutDataTypeStr=double  PortDimensions=1
  SOC / 0..1 : Outport  Port=3  OutDataTypeStr=double  PortDimensions=1
  SOHc / 0..1 : Outport  Port=4  OutDataTypeStr=double  PortDimensions=1
  T_sim / °C : Outport  Port=5  OutDataTypeStr=double  PortDimensions=1
  Generated Heat / W : Outport  Port=6  OutDataTypeStr=double  PortDimensions=1
  SOHr / 1 : Outport  Port=7  OutDataTypeStr=double  PortDimensions=1
  Power_sim / W : Outport  Port=8  OutDataTypeStr=double  PortDimensions=1
  total_Ah : Outport  Port=9
  wires:
  __UniqueInportName__1__/1 -> Current / A/1  "I"
  __UniqueInportName__2__/1 -> Voltage / V/1  "U"
  __UniqueInportName__3__/1 -> SOC / 0..1/1
  __UniqueInportName__4__/1 -> SOHc / 0..1/1  "SOHc"
  __UniqueInportName__5__/1 -> T_sim / °C/1  "simulated Temperature"
  __UniqueInportName__6__/1 -> Generated Heat / W/1
  __UniqueInportName__7__/1 -> SOHr / 1/1  "SOHr"
  __UniqueInportName__8__/1 -> Power_sim / W/1
  __UniqueInportName__9__/1 -> total_Ah/1  "total_Ah"

== system empirical_cell_twaice_balancing/Cell 2/SOC coloumb counting1/__InputSSForSFun__ ==
  SOC_init : Inport
  T_init : Inport  Port=2
  I [A] : Inport  Port=3
  SOHc : Inport  Port=4
  Tcell : Inport  Port=5
  __UniqueOutportName__1__ : Outport  VectorParamsAs1DForOutWhenUnconnected=off
  __UniqueOutportName__2__ : Outport  Port=2  VectorParamsAs1DForOutWhenUnconnected=off
  __UniqueOutportName__3__ : Outport  Port=3  VectorParamsAs1DForOutWhenUnconnected=off
  __UniqueOutportName__4__ : Outport  Port=4  VectorParamsAs1DForOutWhenUnconnected=off
  __UniqueOutportName__5__ : Outport  Port=5  VectorParamsAs1DForOutWhenUnconnected=off
  wires:
  SOC_init/1 -> __UniqueOutportName__1__/1
  T_init/1 -> __UniqueOutportName__2__/1
  I [A]/1 -> __UniqueOutportName__3__/1
  SOHc/1 -> __UniqueOutportName__4__/1
  Tcell/1 -> __UniqueOutportName__5__/1

== system empirical_cell_twaice_balancing/Cell 2/SOC coloumb counting1/__OutputSSForSFun__ ==
  __UniqueInportName__1__ : Inport
  SOC : Outport  VectorParamsAs1DForOutWhenUnconnected=off
  wires:
  __UniqueInportName__1__/1 -> SOC/1

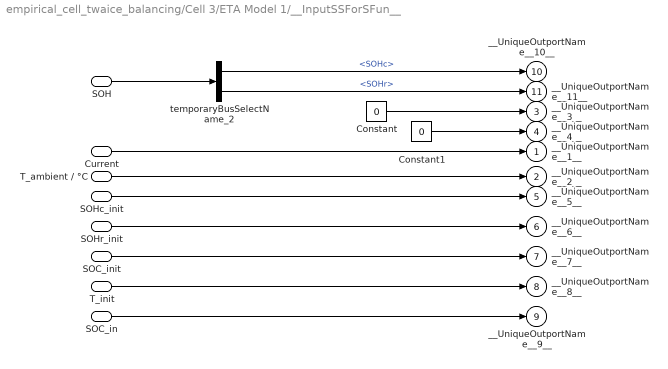
== system empirical_cell_twaice_balancing/Cell 3/ETA Model 1/__InputSSForSFun__ ==
  "Current " : Inport  OutDataTypeStr=double  PortDimensions=1
  T_ambient / °C : Inport  Port=2  OutDataTypeStr=double  PortDimensions=1
  SOHc_init : Inport  Port=3
  SOHr_init : Inport  Port=4
  SOC_init : Inport  Port=5
  T_init : Inport  Port=6
  SOC_in : Inport  Port=7
  SOH : Inport  Port=8
  Constant : Constant  Value=0
  Constant1 : Constant  Value=0
  temporaryBusSelectName_2 : BusSelector  OutputSignals=SOHc,SOHr
  __UniqueOutportName__1__ : Outport  VectorParamsAs1DForOutWhenUnconnected=off
  __UniqueOutportName__2__ : Outport  Port=2  VectorParamsAs1DForOutWhenUnconnected=off
  __UniqueOutportName__3__ : Outport  Port=3  VectorParamsAs1DForOutWhenUnconnected=off
  __UniqueOutportName__4__ : Outport  Port=4  VectorParamsAs1DForOutWhenUnconnected=off
  __UniqueOutportName__5__ : Outport  Port=5  VectorParamsAs1DForOutWhenUnconnected=off
  __UniqueOutportName__6__ : Outport  Port=6  VectorParamsAs1DForOutWhenUnconnected=off
  __UniqueOutportName__7__ : Outport  Port=7  VectorParamsAs1DForOutWhenUnconnected=off
  __UniqueOutportName__8__ : Outport  Port=8  VectorParamsAs1DForOutWhenUnconnected=off
  __UniqueOutportName__9__ : Outport  Port=9  VectorParamsAs1DForOutWhenUnconnected=off
  __UniqueOutportName__10__ : Outport  Port=10  VectorParamsAs1DForOutWhenUnconnected=off
  __UniqueOutportName__11__ : Outport  Port=11  VectorParamsAs1DForOutWhenUnconnected=off
  wires:
  SOH/1 -> temporaryBusSelectName_2/1
  "Current "/1 -> __UniqueOutportName__1__/1
  T_ambient / °C/1 -> __UniqueOutportName__2__/1
  SOHc_init/1 -> __UniqueOutportName__5__/1
  SOHr_init/1 -> __UniqueOutportName__6__/1
  SOC_init/1 -> __UniqueOutportName__7__/1
  T_init/1 -> __UniqueOutportName__8__/1
  SOC_in/1 -> __UniqueOutportName__9__/1
  temporaryBusSelectName_2/1 -> __UniqueOutportName__10__/1  "<SOHc>"
  temporaryBusSelectName_2/2 -> __UniqueOutportName__11__/1  "<SOHr>"
  Constant/1 -> __UniqueOutportName__3__/1
  Constant1/1 -> __UniqueOutportName__4__/1

== system empirical_cell_twaice_balancing/Cell 3/ETA Model 1/__OutputSSForSFun__ ==
  __UniqueInportName__1__ : Inport
  __UniqueInportName__2__ : Inport  Port=2
  __UniqueInportName__3__ : Inport  Port=3
  __UniqueInportName__4__ : Inport  Port=4
  __UniqueInportName__5__ : Inport  Port=5
  __UniqueInportName__6__ : Inport  Port=6
  __UniqueInportName__7__ : Inport  Port=7
  __UniqueInportName__8__ : Inport  Port=8
  __UniqueInportName__9__ : Inport  Port=9
  Current / A : Outport  OutDataTypeStr=double  PortDimensions=1
  Voltage / V : Outport  Port=2  OutDataTypeStr=double  PortDimensions=1
  SOC / 0..1 : Outport  Port=3  OutDataTypeStr=double  PortDimensions=1
  SOHc / 0..1 : Outport  Port=4  OutDataTypeStr=double  PortDimensions=1
  T_sim / °C : Outport  Port=5  OutDataTypeStr=double  PortDimensions=1
  Generated Heat / W : Outport  Port=6  OutDataTypeStr=double  PortDimensions=1
  SOHr / 1 : Outport  Port=7  OutDataTypeStr=double  PortDimensions=1
  Power_sim / W : Outport  Port=8  OutDataTypeStr=double  PortDimensions=1
  total_Ah : Outport  Port=9
  wires:
  __UniqueInportName__1__/1 -> Current / A/1  "I"
  __UniqueInportName__2__/1 -> Voltage / V/1  "U"
  __UniqueInportName__3__/1 -> SOC / 0..1/1
  __UniqueInportName__4__/1 -> SOHc / 0..1/1  "SOHc"
  __UniqueInportName__5__/1 -> T_sim / °C/1  "simulated Temperature"
  __UniqueInportName__6__/1 -> Generated Heat / W/1
  __UniqueInportName__7__/1 -> SOHr / 1/1  "SOHr"
  __UniqueInportName__8__/1 -> Power_sim / W/1
  __UniqueInportName__9__/1 -> total_Ah/1  "total_Ah"

== system empirical_cell_twaice_balancing/Cell 3/SOC coloumb counting1/__InputSSForSFun__ ==
  SOC_init : Inport
  T_init : Inport  Port=2
  I [A] : Inport  Port=3
  SOHc : Inport  Port=4
  Tcell : Inport  Port=5
  __UniqueOutportName__1__ : Outport  VectorParamsAs1DForOutWhenUnconnected=off
  __UniqueOutportName__2__ : Outport  Port=2  VectorParamsAs1DForOutWhenUnconnected=off
  __UniqueOutportName__3__ : Outport  Port=3  VectorParamsAs1DForOutWhenUnconnected=off
  __UniqueOutportName__4__ : Outport  Port=4  VectorParamsAs1DForOutWhenUnconnected=off
  __UniqueOutportName__5__ : Outport  Port=5  VectorParamsAs1DForOutWhenUnconnected=off
  wires:
  SOC_init/1 -> __UniqueOutportName__1__/1
  T_init/1 -> __UniqueOutportName__2__/1
  I [A]/1 -> __UniqueOutportName__3__/1
  SOHc/1 -> __UniqueOutportName__4__/1
  Tcell/1 -> __UniqueOutportName__5__/1

== system empirical_cell_twaice_balancing/Cell 3/SOC coloumb counting1/__OutputSSForSFun__ ==
  __UniqueInportName__1__ : Inport
  SOC : Outport  VectorParamsAs1DForOutWhenUnconnected=off
  wires:
  __UniqueInportName__1__/1 -> SOC/1

== system empirical_cell_twaice_balancing/Cell 4/ETA Model 1/__InputSSForSFun__ ==
  "Current " : Inport  OutDataTypeStr=double  PortDimensions=1
  T_ambient / °C : Inport  Port=2  OutDataTypeStr=double  PortDimensions=1
  SOHc_init : Inport  Port=3
  SOHr_init : Inport  Port=4
  SOC_init : Inport  Port=5
  T_init : Inport  Port=6
  SOC_in : Inport  Port=7
  SOH : Inport  Port=8
  Constant : Constant  Value=0
  Constant1 : Constant  Value=0
  temporaryBusSelectName_2 : BusSelector  OutputSignals=SOHc,SOHr
  __UniqueOutportName__1__ : Outport  VectorParamsAs1DForOutWhenUnconnected=off
  __UniqueOutportName__2__ : Outport  Port=2  VectorParamsAs1DForOutWhenUnconnected=off
  __UniqueOutportName__3__ : Outport  Port=3  VectorParamsAs1DForOutWhenUnconnected=off
  __UniqueOutportName__4__ : Outport  Port=4  VectorParamsAs1DForOutWhenUnconnected=off
  __UniqueOutportName__5__ : Outport  Port=5  VectorParamsAs1DForOutWhenUnconnected=off
  __UniqueOutportName__6__ : Outport  Port=6  VectorParamsAs1DForOutWhenUnconnected=off
  __UniqueOutportName__7__ : Outport  Port=7  VectorParamsAs1DForOutWhenUnconnected=off
  __UniqueOutportName__8__ : Outport  Port=8  VectorParamsAs1DForOutWhenUnconnected=off
  __UniqueOutportName__9__ : Outport  Port=9  VectorParamsAs1DForOutWhenUnconnected=off
  __UniqueOutportName__10__ : Outport  Port=10  VectorParamsAs1DForOutWhenUnconnected=off
  __UniqueOutportName__11__ : Outport  Port=11  VectorParamsAs1DForOutWhenUnconnected=off
  wires:
  SOH/1 -> temporaryBusSelectName_2/1
  "Current "/1 -> __UniqueOutportName__1__/1
  T_ambient / °C/1 -> __UniqueOutportName__2__/1
  SOHc_init/1 -> __UniqueOutportName__5__/1
  SOHr_init/1 -> __UniqueOutportName__6__/1
  SOC_init/1 -> __UniqueOutportName__7__/1
  T_init/1 -> __UniqueOutportName__8__/1
  SOC_in/1 -> __UniqueOutportName__9__/1
  temporaryBusSelectName_2/1 -> __UniqueOutportName__10__/1  "<SOHc>"
  temporaryBusSelectName_2/2 -> __UniqueOutportName__11__/1  "<SOHr>"
  Constant/1 -> __UniqueOutportName__3__/1
  Constant1/1 -> __UniqueOutportName__4__/1

== system empirical_cell_twaice_balancing/Cell 4/ETA Model 1/__OutputSSForSFun__ ==
  __UniqueInportName__1__ : Inport
  __UniqueInportName__2__ : Inport  Port=2
  __UniqueInportName__3__ : Inport  Port=3
  __UniqueInportName__4__ : Inport  Port=4
  __UniqueInportName__5__ : Inport  Port=5
  __UniqueInportName__6__ : Inport  Port=6
  __UniqueInportName__7__ : Inport  Port=7
  __UniqueInportName__8__ : Inport  Port=8
  __UniqueInportName__9__ : Inport  Port=9
  Current / A : Outport  OutDataTypeStr=double  PortDimensions=1
  Voltage / V : Outport  Port=2  OutDataTypeStr=double  PortDimensions=1
  SOC / 0..1 : Outport  Port=3  OutDataTypeStr=double  PortDimensions=1
  SOHc / 0..1 : Outport  Port=4  OutDataTypeStr=double  PortDimensions=1
  T_sim / °C : Outport  Port=5  OutDataTypeStr=double  PortDimensions=1
  Generated Heat / W : Outport  Port=6  OutDataTypeStr=double  PortDimensions=1
  SOHr / 1 : Outport  Port=7  OutDataTypeStr=double  PortDimensions=1
  Power_sim / W : Outport  Port=8  OutDataTypeStr=double  PortDimensions=1
  total_Ah : Outport  Port=9
  wires:
  __UniqueInportName__1__/1 -> Current / A/1  "I"
  __UniqueInportName__2__/1 -> Voltage / V/1  "U"
  __UniqueInportName__3__/1 -> SOC / 0..1/1
  __UniqueInportName__4__/1 -> SOHc / 0..1/1  "SOHc"
  __UniqueInportName__5__/1 -> T_sim / °C/1  "simulated Temperature"
  __UniqueInportName__6__/1 -> Generated Heat / W/1
  __UniqueInportName__7__/1 -> SOHr / 1/1  "SOHr"
  __UniqueInportName__8__/1 -> Power_sim / W/1
  __UniqueInportName__9__/1 -> total_Ah/1  "total_Ah"

== system empirical_cell_twaice_balancing/Cell 4/SOC coloumb counting1/__InputSSForSFun__ ==
  SOC_init : Inport
  T_init : Inport  Port=2
  I [A] : Inport  Port=3
  SOHc : Inport  Port=4
  Tcell : Inport  Port=5
  __UniqueOutportName__1__ : Outport  VectorParamsAs1DForOutWhenUnconnected=off
  __UniqueOutportName__2__ : Outport  Port=2  VectorParamsAs1DForOutWhenUnconnected=off
  __UniqueOutportName__3__ : Outport  Port=3  VectorParamsAs1DForOutWhenUnconnected=off
  __UniqueOutportName__4__ : Outport  Port=4  VectorParamsAs1DForOutWhenUnconnected=off
  __UniqueOutportName__5__ : Outport  Port=5  VectorParamsAs1DForOutWhenUnconnected=off
  wires:
  SOC_init/1 -> __UniqueOutportName__1__/1
  T_init/1 -> __UniqueOutportName__2__/1
  I [A]/1 -> __UniqueOutportName__3__/1
  SOHc/1 -> __UniqueOutportName__4__/1
  Tcell/1 -> __UniqueOutportName__5__/1
